simulink model "FinalProject"  (R2012b)
settings: Solver=ode1  StartTime=0.0  StopTime=inf  FixedStep=0.002  RelTol=1e-3
undefined symbols (not defined in the file or in its folder): HIL, qc_get_step_size
libraries: simulink x6, quarc_library x6
settings Model: SimulationMode=external  ExtModeTrigDuration=5000  Creator=runkunwang  LastModifiedBy=runkunwang
settings SolverCC: PositivePriorityOrder=on
settings RTWCC: SystemTargetFile=quarc_win64.tlc  TemplateMakefile=quarc_default_tmf  Description=QUARC Win64 Target  ProcessScript=quarc_win64_make_rtw_hook
settings STFCustomTargetCC: TargetPreCompLibLocation=C:\PROGRA~3\QUARC\lib\2012b\win64\release  CodeReplacementLibrary=ANSI_C  GeneratePreprocessorConditionals=Disable all  CombineOutputUpdateFcns=on  GRTInterface=off  SystemTargetFile=quarc_win64.tlc
settings GRTTargetCC: TargetPreCompLibLocation=C:\PROGRA~3\QUARC\lib\2012b\win64\release  ParMdlRefBuildCompliant=off  CompOptLevelCompliant=off  ConcurrentExecutionCompliant=off  MatFileLogging=off  ExtMode=on  ExtModeMexFile=quarc_comm

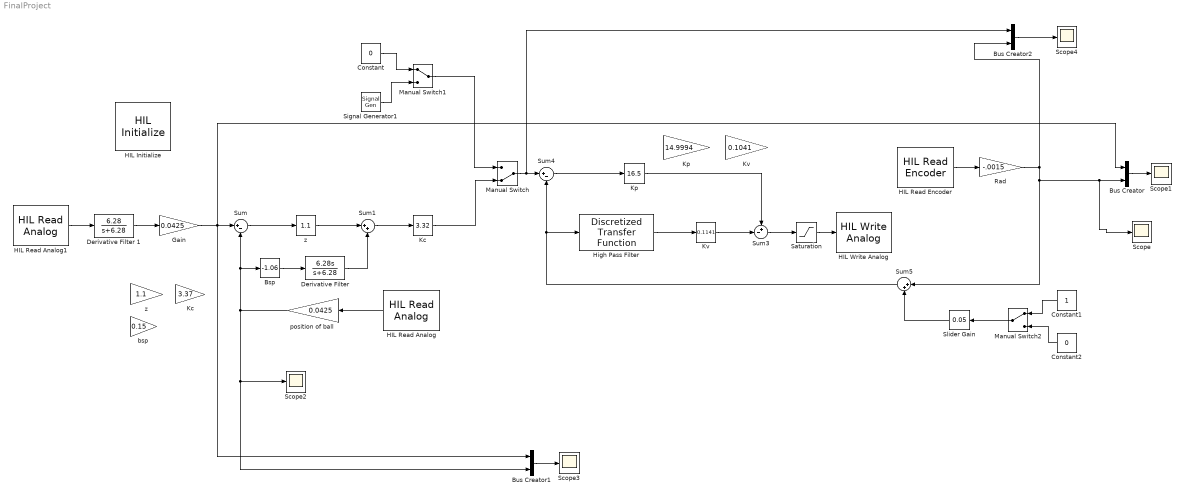
== system FinalProject ==
  Bsp : simulink/Math Operations/Slider Gain  low=-1.5  gain=-1.06  high=0
  Bus Creator : BusCreator  Inputs=2
  Bus Creator1 : BusCreator  Inputs=2
  Bus Creator2 : BusCreator  Inputs=2
  Constant : Constant  Value=0
  Constant1 : Constant
  Constant2 : Constant  Value=0
  "Derivative Filter " : TransferFcn  Numerator=[6.28 0]  Denominator=[1 6.28]
  Derivative Filter 1 : TransferFcn  Numerator=[6.28]  Denominator=[1 6.28]
  Gain : Gain  Gain=0.0425
  HIL Initialize : quarc_library/Data Acquisition/Generic/Configuration/HIL Initialize  Priority=-99  object_name=HIL-1  board_type=q2_usb  board_number=0  board_options=d0=digital;d1=digital;led=auto;update_rate=normal;decimation=1  exclusive=off  active=off  hardware_clocks=[0]  clock_modes=[]  initial_clock_frequencies=[]  set_clock_params_at_start=off  set_clock_params_at_switch_in=off  set_clock_frequencies_at_start=off  set_clock_frequencies_at_switch_in=off  analog_input_channels=[0:1]  analog_input_maximums=10  analog_input_minimums=-10  set_analog_input_params_at_start=on  set_analog_input_params_at_switch_in=off  analog_output_channels=[0:1]  analog_output_maximums=10  analog_output_minimums=-10  initial_analog_outputs=[0]  final_analog_outputs=[0]  watchdog_analog_outputs=0  set_analog_output_params_at_start=on  set_analog_output_params_at_switch_in=off  set_analog_outputs_at_start=on  set_analog_outputs_at_switch_in=off  set_analog_outputs_at_terminate=on  set_analog_outputs_at_switch_out=off  set_analog_outputs_on_watchdog=off  digital_input_channels=[]  digital_output_channels=[]  digital_output_configuration=[]  initial_digital_outputs=[1]  final_digital_outputs=[1]  watchdog_digital_outputs=[1]  set_digital_output_params_at_start=off  set_digital_output_params_at_switch_in=off  set_digital_outputs_at_start=on  set_digital_outputs_at_switch_in=off  set_digital_outputs_at_terminate=on  set_digital_outputs_at_switch_out=off  set_digital_outputs_on_watchdog=off  encoder_channels=[0:1]  quadrature=[4]  encoder_filter_frequency=[]  initial_encoder_counts=[0]  set_encoder_params_at_start=on  set_encoder_params_at_switch_in=off  set_encoder_counts_at_start=on  set_encoder_counts_at_switch_in=off  pwm_channels=[]  pwm_modes=[0]  pwm_frequency=1/0.020  pwm_configuration=[]  pwm_alignment=[]  pwm_polarity=[]  pwm_leading_deadband=[]  pwm_trailing_deadband=[]  initial_pwm_outputs=[0]  final_pwm_outputs=[0]  watchdog_pwm_outputs=[0]  set_pwm_params_at_start=on  set_pwm_params_at_switch_in=off  set_pwm_outputs_at_start=on  set_pwm_outputs_at_switch_in=off  set_pwm_outputs_at_terminate=on  set_pwm_outputs_at_switch_out=off  set_pwm_outputs_on_watchdog=off  other_output_channels=[]  initial_other_outputs=[]  final_other_outputs=[]  watchdog_other_outputs=[]  set_other_outputs_at_start=off  set_other_outputs_at_switch_in=off  set_other_outputs_at_terminate=off  set_other_outputs_at_switch_out=off  set_other_outputs_on_watchdog=off
  HIL Read Analog : quarc_library/Data Acquisition/Generic/Immediate I//O/HIL Read Analog  object_name=HIL-1  channels=0  sample_time=qc_get_step_size  active=on  vector_output=off
  HIL Read Analog1 : quarc_library/Data Acquisition/Generic/Immediate I//O/HIL Read Analog  object_name=HIL-1  channels=1  sample_time=qc_get_step_size  active=on  vector_output=off
  HIL Read Encoder : quarc_library/Data Acquisition/Generic/Immediate I//O/HIL Read Encoder  object_name=HIL-1  channels=0  sample_time=qc_get_step_size  active=on  vector_output=off  data_type_mode=Inherit via back propagation  data_type=double
  HIL Write Analog : quarc_library/Data Acquisition/Generic/Immediate I//O/HIL Write Analog  object_name=HIL-1  channels=0  sample_time=-1  active=off  vector_input=off
  High Pass Filter : quarc_library/Discrete/Discretized Transfer Function  num=[24674 0]  den=[1 141.3717 24674]  method=tustin  Ts=qc_get_step_size
  Kc : simulink/Math Operations/Slider Gain  low=0  gain=3.32  high=7
  "Kc " : Gain  Gain=3.37
  Kp : Gain  Gain=14.9994
  "Kp " : simulink/Math Operations/Slider Gain  low=12  gain=16.5  high=18
  Kv : Gain  Gain=0.1041
  "Kv " : simulink/Math Operations/Slider Gain  low=0  gain=0.1141  high=0.3
  Manual Switch : ManualSwitch  CurrentSetting=0
  Manual Switch1 : ManualSwitch
  Manual Switch2 : ManualSwitch
  Rad : Gain  Gain=-.0015
  Saturation : Saturate  UpperLimit=10  LowerLimit=-10
  Scope{,1..4} (5 alike) : Scope
      Scope settings: YMin=-0.5  YMax=0.25  SaveName=PracMech
      Scope1 settings: YMin=-0.25  YMax=3.5
      Scope3 settings: YMin=-0.225  YMax=0.225  SaveName=PracMechExp  MaxDataPoints=10000
      Scope4 settings: YMin=-0.2  YMax=1.8  SaveName=ScopeData3
  Signal Generator1 : SignalGenerator  WaveForm=square  Frequency=0.25
  Slider Gain : simulink/Math Operations/Slider Gain  low=-4  gain=0.05  high=1
  Sum : Sum  Inputs=|+-
  Sum1 : Sum  Inputs=|++
  Sum3 : Sum  Inputs=+-|
  Sum4 : Sum  Inputs=|+-
  Sum5 : Sum  Inputs=|++
  "bsp " : Gain  Gain=0.15
  "position of ball " : Gain  Gain=0.0425
  "z " : Gain  Gain=1.1
  "z " : simulink/Math Operations/Slider Gain  low=0  gain=1.1  high=6.0415
  wires:
  Gain/1 -> Bus Creator1/1, Bus Creator/1, Sum/1
  HIL Read Encoder/1 -> Rad/1
  "z "/1 -> Sum1/1
  Sum/1 -> "z "/1
  Sum1/1 -> Kc/1
  Bus Creator/1 -> Scope1/1
  "Derivative Filter "/1 -> Sum1/2
  Bsp/1 -> "Derivative Filter "/1
  Rad/1 -> Sum5/1, Bus Creator/2, Scope/1, Bus Creator2/2
  "Kp "/1 -> Sum3/1
  "Kv "/1 -> Sum3/2
  Sum4/1 -> "Kp "/1
  Manual Switch/1 -> Bus Creator2/1, Sum4/1
  Manual Switch1/1 -> Manual Switch/1
  Kc/1 -> Manual Switch/2
  Saturation/1 -> HIL Write Analog/1
  Sum3/1 -> Saturation/1
  Sum5/1 -> High Pass Filter/1, Sum4/2
  Slider Gain/1 -> Sum5/2
  HIL Read Analog/1 -> "position of ball "/1
  "position of ball "/1 -> Bus Creator1/2, Scope2/1, Bsp/1, Sum/2
  Bus Creator1/1 -> Scope3/1
  Constant/1 -> Manual Switch1/1
  Signal Generator1/1 -> Manual Switch1/2
  Bus Creator2/1 -> Scope4/1
  High Pass Filter/1 -> "Kv "/1
  Manual Switch2/1 -> Slider Gain/1
  Constant1/1 -> Manual Switch2/1
  Constant2/1 -> Manual Switch2/2
  HIL Read Analog1/1 -> Derivative Filter 1/1
  Derivative Filter 1/1 -> Gain/1
